simulink model "RateAdaption"  (R2022a)
settings: Solver=FixedStepAuto  StartTime=0.0  StopTime=10.0  FixedStep=1e-3  RelTol=1e-3  EnableMultiTasking=on
libraries: frdmk64flib x1, dspstat3 x1
settings Model: ExtModeTrigDuration=5  Creator=kemij  LastModifiedBy=Motz
settings OptimizationCC: EnhancedBackFolding=on  PassReuseOutputArgsAs=Individual arguments  ZeroExternalMemoryAtStartup=off  ZeroInternalMemoryAtStartup=off  MaxStackSize=64  OptimizeBlockOrder=speed  DifferentSizesBufferReuse=on  OptimizationCustomize=off  EfficientTunableParamExpr=on
settings DebuggingCC: ParameterTunabilityLossMsg=error
settings HardwareCC: ProdBitPerPointer=32  ProdBitPerSizeT=32  ProdBitPerPtrDiffT=32  ProdLargestAtomicInteger=Long  ProdLargestAtomicFloat=Double  ProdWordSize=32  ProdHWDeviceType=ARM Compatible->ARM Cortex
settings SFSimCC: MATLABDynamicMemAlloc=off
settings RTWCC: SystemTargetFile=ert.tlc  HardwareBoard=NXP FRDM-K64F  TLCOptions="-aInlineSetEventsForThisBaseRateFcn=TLC_FALSE -aSuppressMultiTaskScheduler=TLC_FALSE  -aRateBasedStepFcn=0"  TemplateMakefile=ert_default_tmf  Toolchain=GNU Tools for ARM Embedded Processors
settings CodeAppCC: ForceParamTrailComments=on  IgnoreCustomStorageClasses=off  OperatorAnnotations=on  SimulinkDataObjDesc=on  SFDataObjDesc=on  InsertBlockDesc=on
settings ERTTargetCC: ExtModeTransport=4  ExtModeMexFile=sendToCommService

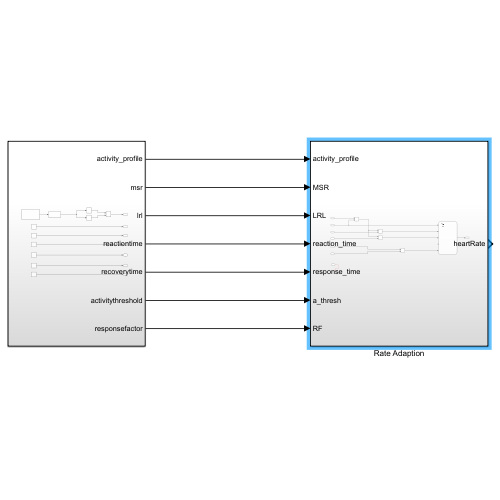
[thumbnail: Simulink's stored preview of the top-level diagram]
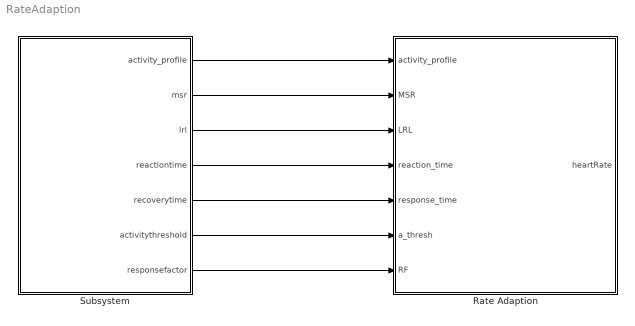
== system RateAdaption ==
  Rate Adaption : Subsystem
  Subsystem : Subsystem
  wires:
  Subsystem/1(activity_profile) -> Rate Adaption/1(activity_profile)
  Subsystem/2(msr) -> Rate Adaption/2(MSR)
  Subsystem/3(lrl) -> Rate Adaption/3(LRL)
  Subsystem/4(reactiontime) -> Rate Adaption/4(reaction_time)
  Subsystem/5(recoverytime) -> Rate Adaption/5(response_time)
  Subsystem/6(activitythreshold) -> Rate Adaption/6(a_thresh)
  Subsystem/7(responsefactor) -> Rate Adaption/7(RF)

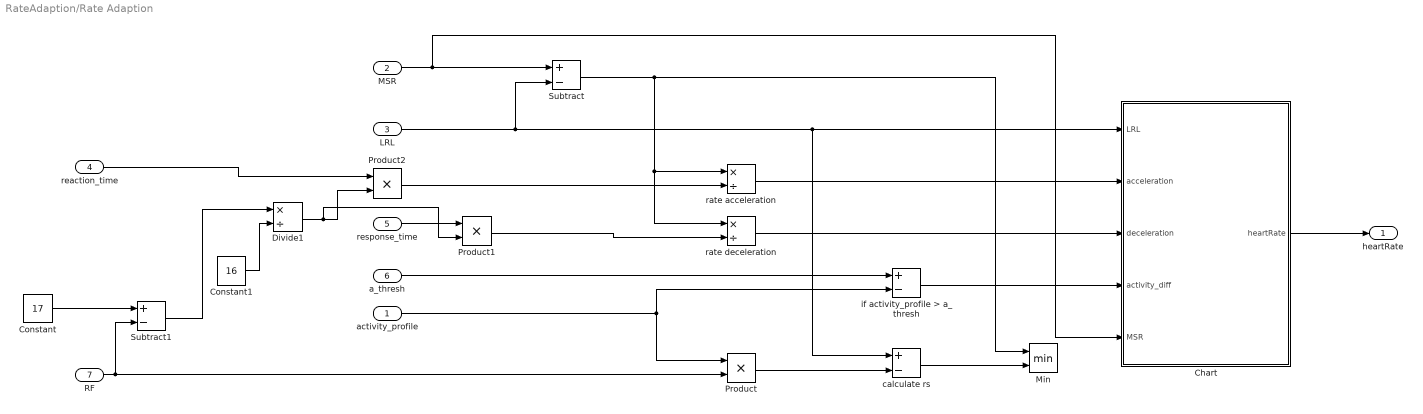
== system RateAdaption/Rate Adaption ==
  activity_profile : Inport
  MSR : Inport  Port=2
  LRL : Inport  Port=3
  reaction_time : Inport  Port=4
  response_time : Inport  Port=5
  a_thresh : Inport  Port=6
  RF : Inport  Port=7
  Chart : Stateflow chart  TreatAsAtomicUnit=on
      settings: PortSchema="{\"entries\":[{\"content\":{\"sides\":[{\"content\":{\"connectorIds\":[\"In5\",\"In1\",\"In3\",\"In2\",\"In4\"]},\"type\":\"ConnectorPlacement.EquallySpacedRectSide\",\"uuid\":\"f1bfb65c-a3e0-488b-a51c-ed381b80a0d3\"},{\"content\":{\"connectorIds\":[\"Out1\"],\"side\":\"RIGHT\"},\"type\":\"ConnectorPlacement.EquallySpacedRectSide\",\"uuid\":\"38293472-2491-4ffe-ba83-6a5f72f7d4c8\"},{\"content\":{\"connectorIds\":[],\"side\":\"TOP\"},\"type\":\"ConnectorPlacement.EquallySpacedRectSide\",\"uuid\":\"d4d219f0-2dab-436b-b9c2-781e051d4797\"}]},\"type\":\"ConnectorPlacement.EquallySpacedConnector\",\"uuid\":\"faf9de58-f900-4f39-b014-8d2778c5d5cd\"}],\"packageUris\":[\"http://schema.mathworks.com/mf0/Connector/R2020b\"],\"version\":\"1.0\"}"
  Constant : Constant  Value=17
  Constant1 : Constant  Value=16
  Divide1 : Product  Inputs=*/
  Min : MinMax  Inputs=2
  Product : Product
  Product1 : Product
  Product2 : Product
  Subtract : Sum  Inputs=+-
  Subtract1 : Sum  Inputs=+-
  calculate rs : Sum  Inputs=+-
  if activity_profile > a_thresh : Sum  Inputs=+-
  rate acceleration : Product  Inputs=*/
  rate deceleration : Product  Inputs=*/
  heartRate : Outport
  wires:
  MSR/1 -> Chart/4(MSR), Subtract/1
  Chart/1(heartRate) -> heartRate/1
  LRL/1 -> calculate rs/1, Chart/5(LRL), Subtract/2
  Subtract/1 -> rate deceleration/1, rate acceleration/1, Min/1
  RF/1 -> Subtract1/2, Product/2
  rate acceleration/1 -> Chart/1(acceleration)
  rate deceleration/1 -> Chart/3(deceleration)
  if activity_profile > a_thresh/1 -> Chart/2(activity_diff)
  a_thresh/1 -> if activity_profile > a_thresh/1
  activity_profile/1 -> Product/1, if activity_profile > a_thresh/2
  Product/1 -> calculate rs/2
  calculate rs/1 -> Min/2
  Product2/1 -> rate acceleration/2
  Constant/1 -> Subtract1/1
  Subtract1/1 -> Divide1/1
  Constant1/1 -> Divide1/2
  reaction_time/1 -> Product2/1
  Divide1/1 -> Product2/2, Product1/2
  response_time/1 -> Product1/1
  Product1/1 -> rate deceleration/2

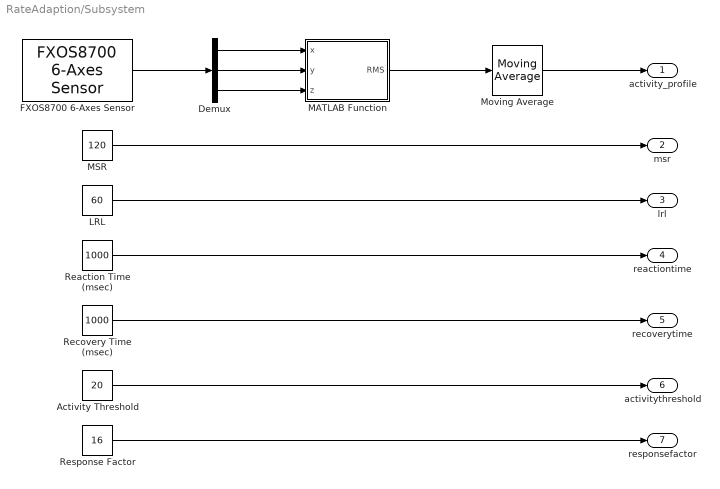
== system RateAdaption/Subsystem ==
  Activity Threshold : Constant  Value=20
  Demux : Demux  Outputs=3
  FXOS8700 6-Axes Sensor : frdmk64flib/FXOS8700 6-Axes Sensor  Activesensor=Accelerometer only  ODR=800Hz  HybridODR=400Hz  Accelfullrange=-4g to +4g  SampleTime=-1
  LRL : Constant  Value=60
  MATLAB Function : MATLAB Function  TreatAsAtomicUnit=on
  MSR : Constant  Value=120
  Moving Average : dspstat3/Moving Average  Method=Sliding window  ForgettingFactorPort=off  SpecifyWindowLength=on  WindowLength=4  ForgettingFactor=0.9  SimulateUsing=Code generation
  Reaction Time (msec) : Constant  Value=1000
  Recovery Time (msec) : Constant  Value=1000
  Response Factor : Constant  Value=16
  activity_profile : Outport
  msr : Outport  Port=2
  lrl : Outport  Port=3
  reactiontime : Outport  Port=4
  recoverytime : Outport  Port=5
  activitythreshold : Outport  Port=6
  responsefactor : Outport  Port=7
  wires:
  Moving Average/1 -> activity_profile/1
  MSR/1 -> msr/1
  LRL/1 -> lrl/1
  Reaction Time (msec)/1 -> reactiontime/1
  Recovery Time (msec)/1 -> recoverytime/1
  Activity Threshold/1 -> activitythreshold/1
  Response Factor/1 -> responsefactor/1
  Demux/3 -> MATLAB Function/3(z)
  Demux/2 -> MATLAB Function/2(y)
  MATLAB Function/1(RMS) -> Moving Average/1
  Demux/1 -> MATLAB Function/1(x)
  FXOS8700 6-Axes Sensor/1 -> Demux/1

== matlab function RateAdaption/Subsystem/MATLAB Function ==
  data: x input; RMS output; y input; z input
function RMS = calc_RMS(x,y,z)

RMS = sqrt((x^2 + y^2 + z^2)/3.0);

== stateflow chart RateAdaption/Rate Adaption/Chart ==
  state IncreaseHeartRate
    during:
    activity_time = elapsed(msec)
    heartRate = heartRate + acceleration*activity_time
  state HOLDSensorRate
    during:
    heartRate = MSR
  state IDLE
    entry:
    heartRate = LRL
    activity_time = 0
    zero_activity_time = 0
  state ActivitySensed
    %activity has been sensed
  state HOLDLRL
    during:
    heartRate = LRL
  state DecreaseHeartRate
    % decrease rate until there is zero activity (0 bpm)
    during:
    zero_activity_time = elapsed(msec)
    heartRate = heartRate - deceleration*zero_activity_time
  (junction 15) -> IncreaseHeartRate [order 1] : [heartRate + acceleration*activity_time <MSR]
  IncreaseHeartRate -> (junction 26) : [heartRate==MSR || activity_diff<=0 ]
  ActivitySensed -> (junction 15) [order 2] : [activity_diff > 0]
  (junction 15) -> HOLDSensorRate [order 2] : [heartRate + acceleration*activity_time >= MSR]
  HOLDSensorRate -> (junction 26) : [activity_diff<=0]
  (default) -> IDLE
  IDLE -> ActivitySensed
  (junction 26) -> ActivitySensed
  HOLDLRL -> (junction 26) : [activity_diff>0]
  DecreaseHeartRate -> (junction 26) : [activity_diff>0||heartRate==LRL]
  ActivitySensed -> (junction 16) [order 1] : [activity_diff <= 0]
  (junction 16) -> HOLDLRL [order 2] : [heartRate - deceleration*zero_activity_time <= LRL]
  (junction 16) -> DecreaseHeartRate [order 1] : [heartRate - deceleration*zero_activity_time > LRL]
  data: acceleration input; activity_diff input; deceleration input; MSR input; activity_time local; LRL input; zero_activity_time local; heartRate output
